simulink model "rtwdemo_PCG_Eval_P5"  (Simulink 7.6)
settings: Solver=FixedStepDiscrete  SolverMode=SingleTasking  StartTime=0.0  StopTime=2  FixedStep=.001  MaxStep=10  RelTol=1e-3
PostLoadFcn:
  | if (exist('PCG_Demo_5_data','file'))
  |    load PCG_Demo_5_data;
  | else
  |    % Load Data Objects
  |    RTWDemos.PCG_Eval_Base_Data_Stage_5;
  | end
libraries: rtwdemo_pi_controller x2, rtwdemo_SimpleSchedModel x1
CloseFcn:
  | rtwprivate ssgencode ModelCloseRequest rtwdemo_PCG_Eval_P1
settings Model: Creator=The MathWorks Inc.  ExtModeAutoUpdateStatusClock=off
settings SolverCC: InsertRTBMode=Auto
settings DataIOCC: LimitDataPoints=off  SaveFormat=StructureWithTime  SaveOutput=off  SaveTime=off
settings OptimizationCC: InlineParams=on  LocalBlockOutputs=off  StateBitsets=on  DataBitsets=on  UseTempVars=on  ZeroExternalMemoryAtStartup=off  ZeroInternalMemoryAtStartup=off  NoFixptDivByZeroProtection=on  EfficientFloat2IntCast=on  EfficientMapNaN2IntZero=off  OptimizeModelRefInitCode=on
settings DebuggingCC: CheckExecutionContextPreStartOutputMsg=on  CheckExecutionContextRuntimeOutputMsg=on  IntegerOverflowMsg=none  InvalidFcnCallConnMsg=warning  BusObjectLabelMismatch=error  RootOutportRequireBusObject=error  ModelReferenceIOMsg=error  ModelReferenceIOMismatchMessage=error  ModelReferenceCSMismatchMessage=error  ModelReferenceDataLoggingMessage=error
settings HardwareCC: ProdHWDeviceType=32-bit Embedded Processor
settings ModelReferenceCC: ModelReferenceNumInstancesAllowed=Single  ModelReferencePassRootInputsByReference=off
settings SFSimCC: SimCustomHeaderCode="#include \"ThrottleBus.h\""  SimUserIncludeDirs="\"$matlabroot$\\toolbox\\rtw\\rtwdemos\\EmbeddedCoderOverview\\\""  SimParseCustomCode=off
settings RTWCC: SystemTargetFile=ert.tlc  GenCodeOnly=on  TemplateMakefile=ert_default_tmf  PostCodeGenCommand=packNGo(buildInfo)  Description=Real-Time Workshop Embedded Coder (no auto configuration)  GenerateReport=on  ProcessScript=ert_make_rtw_hook  CustomHeaderCode="#include \"ThrottleBus.h\""  IncludeHyperlinkInReport=on
settings RTWCC: CustomInclude=|
  | "$matlabroot$\toolbox\rtw\rtwdemos\EmbeddedCoderOverview\stage_5_files\"
  | "$matlabroot$\toolbox\rtw\rtwdemos\EmbeddedCoderOverview\"
settings RTWCC: CustomSource=|
  | defineImportedData.c
  | example_main.c
settings CodeAppCC: ForceParamTrailComments=on  IgnoreCustomStorageClasses=off
settings ERTTargetCC: TargetFcnLib=ansi_tfl_tmw_new.mat  MultiwordLength=2048  GenerateSampleERTMain=on  IncludeMdlTerminateFcn=off  SuppressErrorStatus=on  SupportAbsoluteTime=off  MultiInstanceERTCode=on  SupportNonFinite=off  SupportComplex=off  MultiInstanceErrorCode=None  ERTCustomFileTemplate=example_file_process.tlc  GlobalDataDefinition=InSeparateSourceFile  DataDefinitionFile=eval_data.c  GlobalDataReference=InSeparateHeaderFile  DataReferenceFile=eval_data.h  ConvertIfToSwitch=off  EnableUserReplacementTypes=on  MemSecPackage=Simulink  MemSecDataConstants=MemConst

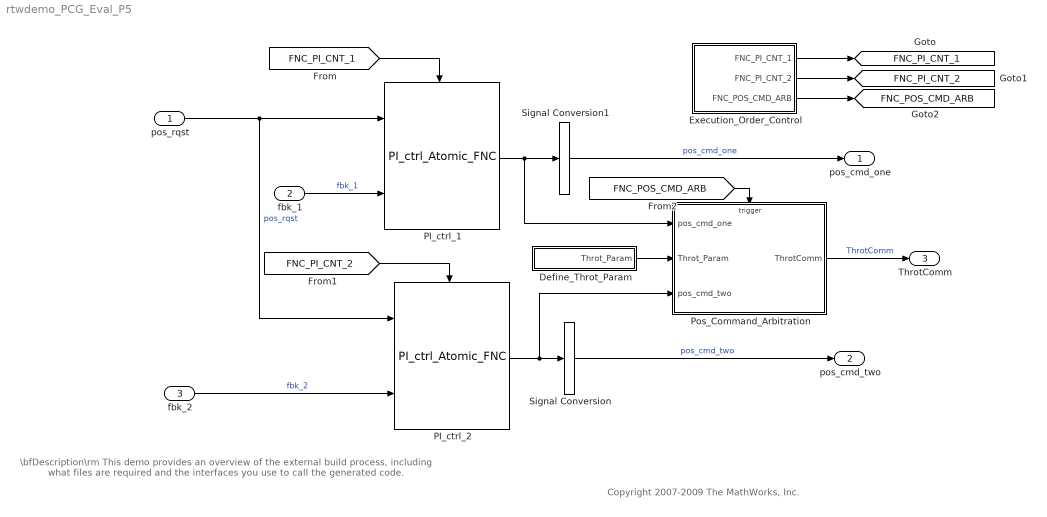
== system rtwdemo_PCG_Eval_P5 ==
  note: Copyright 2007-2009 The MathWorks, Inc.
  note: \bfDescription\rm
      | This demo provides an overview of the external
      | build process, including what files are required
      | and the interfaces you use to call the generated code.
  pos_rqst : Inport
  fbk_1 : Inport  Port=2
  fbk_2 : Inport  Port=3
  Define_Throt_Param : Subsystem  TreatAsAtomicUnit=on  RTWFcnName=Define_Throt_Param
      settings: RTWFcnNameOpts=Use subsystem name  RTWFileNameOpts=Use function name
  Execution_Order_Control : Subsystem  BlockChoice=PI_1_then_PI_2_then_Pos_Cmd_Arb
      settings: AttributesFormatString=%<BlockChoice>  TemplateBlock=rtwdemo_SimpleSchedModel/Execution_Order_Control  MemberBlocks=PI_1_then_PI_2_then_Pos_Cmd_Arb,Pos_Cmd_Arb_then_PI_1_then_PI_2
  PI_ctrl_1 : rtwdemo_pi_controller/PI_ctrl_Atomic_FNC  SystemSampleTime=-1
  PI_ctrl_2 : rtwdemo_pi_controller/PI_ctrl_Atomic_FNC  SystemSampleTime=-1
  Pos_Command_Arbitration : Stateflow chart  TreatAsAtomicUnit=on
      settings: RTWSystemCode=Reusable function  RTWFileNameOpts=Use function name
  Signal Conversion : SignalConversion  ConversionOutput=Contiguous copy  OverrideOpt=on
  Signal Conversion1 : SignalConversion  ConversionOutput=Contiguous copy  OverrideOpt=on
  pos_cmd_one : Outport
  pos_cmd_two : Outport  Port=2
  ThrotComm : Outport  Port=3  OutDataTypeStr=Bus: ThrottleCommands  BusOutputAsStruct=on
  tag scope: FNC_PI_CNT_1=global, FNC_PI_CNT_2=global, FNC_POS_CMD_ARB=global
  wires:
  fbk_1/1 -> PI_ctrl_1/2  "fbk_1"
  fbk_2/1 -> PI_ctrl_2/2  "fbk_2"
  Pos_Command_Arbitration/1(ThrotComm) -> ThrotComm/1  "ThrotComm"
  PI_ctrl_2/1 -> Pos_Command_Arbitration/3(pos_cmd_two), Signal Conversion/1
  PI_ctrl_1/1 -> Pos_Command_Arbitration/1(pos_cmd_one), Signal Conversion1/1
  pos_rqst/1 -> PI_ctrl_1/1, PI_ctrl_2/1  "pos_rqst"
  [FNC_PI_CNT_1] -> PI_ctrl_1/Trigger
  Execution_Order_Control/1(FNC_PI_CNT_1) -> [FNC_PI_CNT_1]
  Execution_Order_Control/2(FNC_PI_CNT_2) -> [FNC_PI_CNT_2]
  Execution_Order_Control/3(FNC_POS_CMD_ARB) -> [FNC_POS_CMD_ARB]
  Define_Throt_Param/1(Throt_Param) -> Pos_Command_Arbitration/2(Throt_Param)
  [FNC_POS_CMD_ARB] -> Pos_Command_Arbitration/Trigger
  [FNC_PI_CNT_2] -> PI_ctrl_2/Trigger
  Signal Conversion/1 -> pos_cmd_two/1  "pos_cmd_two"
  Signal Conversion1/1 -> pos_cmd_one/1  "pos_cmd_one"

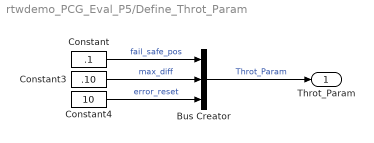
== system rtwdemo_PCG_Eval_P5/Define_Throt_Param ==
  Bus Creator : BusCreator  Inputs=3  OutDataTypeStr=Bus: ThrottleParams  NonVirtualBus=on
  Constant : Constant  Value=.1  OutDataTypeStr=double
  Constant3 : Constant  Value=.10  OutDataTypeStr=double
  Constant4 : Constant  Value=10  OutDataTypeStr=double
  Throt_Param : Outport  OutDataTypeStr=Bus: ThrottleParams
  wires:
  Constant/1 -> Bus Creator/1  "fail_safe_pos"
  Constant3/1 -> Bus Creator/2  "max_diff"
  Constant4/1 -> Bus Creator/3  "error_reset"
  Bus Creator/1 -> Throt_Param/1  "Throt_Param"

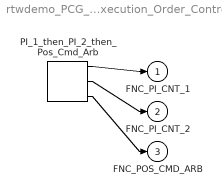
== system rtwdemo_PCG_Eval_P5/Execution_Order_Control ==
  PI_1_then_PI_2_then_Pos_Cmd_Arb : rtwdemo_SimpleSchedModel/PI_1_then_PI_2_then_Pos_Cmd_Arb  SystemSampleTime=-1
  FNC_PI_CNT_1 : Outport
  FNC_PI_CNT_2 : Outport  Port=2
  FNC_POS_CMD_ARB : Outport  Port=3
  wires:
  PI_1_then_PI_2_then_Pos_Cmd_Arb/1 -> FNC_PI_CNT_1/1
  PI_1_then_PI_2_then_Pos_Cmd_Arb/2 -> FNC_PI_CNT_2/1
  PI_1_then_PI_2_then_Pos_Cmd_Arb/3 -> FNC_POS_CMD_ARB/1

== stateflow chart Pos_Command_Arbitration ==
  note: The Stateflow Diagram impliments an if / elseif / else
  note: End of the if structure
  note: The throttle command signals are not in agreement. Enter into fail safe mode
  note: Not in an error mode:
      | The control signal is selected from the input signal that
      | most closly matches the last pass value of the signal
  note: The signals have not been in agreement for a
      | long enough time to exit the failure mode: increment the failure counter
  note: Enough time has passed to exit the failure mode:
      | reset the mode and the counter
  (default) -> (junction 18) : {
      |  ThrotComm.pos_cmd_raw[0] = pos_cmd_one;...
      |  ThrotComm.pos_cmd_raw[1] = pos_cmd_two;
      | }
  (junction 18) -> (junction 10) [order 1] : [abs(pos_cmd_one - pos_cmd_two) > Throt_Param.max_diff]
  (junction 9) -> (junction 11) [order 2]
  (junction 17) -> (junction 12) : {
      | ThrotComm.pos_failure_mode = 0;
      | ThrotComm.err_cnt = 0;
      | }
  (junction 19) -> (junction 16) [order 1] : [ThrotComm.pos_failure_mode > 0]
  (junction 14) -> (junction 15)
  (junction 19) -> (junction 22) [order 2]
  (junction 10) -> (junction 21) : {
      |  ThrotComm.pos_failure_mode = 1;...
      |  ThrotComm.err_cnt = 0;
      |  ThrotComm.pos_cmd_act = Throt_Param.fail_safe_pos;
      | }
  (junction 9) -> (junction 17) [order 1] : [ThrotComm.err_cnt >= Throt_Param.error_reset]
  (junction 18) -> (junction 9) [order 2]
  (junction 16) -> (junction 20) : {
      |  ThrotComm.err_cnt++;
      | }
  (junction 22) -> (junction 14) [order 2] : {
      | ThrotComm.pos_cmd_act = pos_cmd_two;
      | }
  (junction 12) -> (junction 11)
  (junction 22) -> (junction 23) [order 1] : [abs(pos_cmd_one - ThrotComm.pos_cmd_act) < ...
      | abs(pos_cmd_two - ThrotComm.pos_cmd_act)]
  (junction 23) -> (junction 13) : {
      | ThrotComm.pos_cmd_act = pos_cmd_one;
      | }
  (junction 11) -> (junction 19)
  (junction 21) -> (junction 20)
  (junction 20) -> (junction 13)
  (junction 13) -> (junction 14)
  data: pos_cmd_one input double; Throt_Param input Bus: ThrottleParams size=1; pos_cmd_two input double; ThrotComm output Bus: ThrottleCommands size=1; fail_safe_pos local double =.1
  events: FNC_SF_Arbit input FUNCTION_CALL_EVENT
